simulink model "test"  (R2014a)
settings: Solver=VariableStepAuto  StartTime=0.0  StopTime=10.0  RelTol=1e-3
settings Model: Creator=costa  LastModifiedBy=rcostado
settings DataIOCC: LimitDataPoints=off  SaveFormat=Dataset
settings OptimizationCC: SimCompilerOptimization=off
settings DebuggingCC: MergeDetectMultiDrivingBlocksExec=error  SolverPrmCheckMsg=none  FrameProcessingCompatibilityMsg=error
settings HardwareCC: ProdBitPerPointer=64  ProdLargestAtomicFloat=Float  ProdIntDivRoundTo=Zero  ProdEndianess=LittleEndian  ProdWordSize=64  ProdHWDeviceType=Intel->x86-64 (Windows64)
settings ModelReferenceCC: PropagateSignalLabelsOutOfModel=on
settings RTWCC: RTWCompilerOptimization=off
settings ConfigComp: CovMetricSettings=dw  CovHtmlReporting=on  CovSaveCumulativeToWorkspaceVar=on  CovSaveSingleToWorkspaceVar=on  CovExternalEMLEnable=off

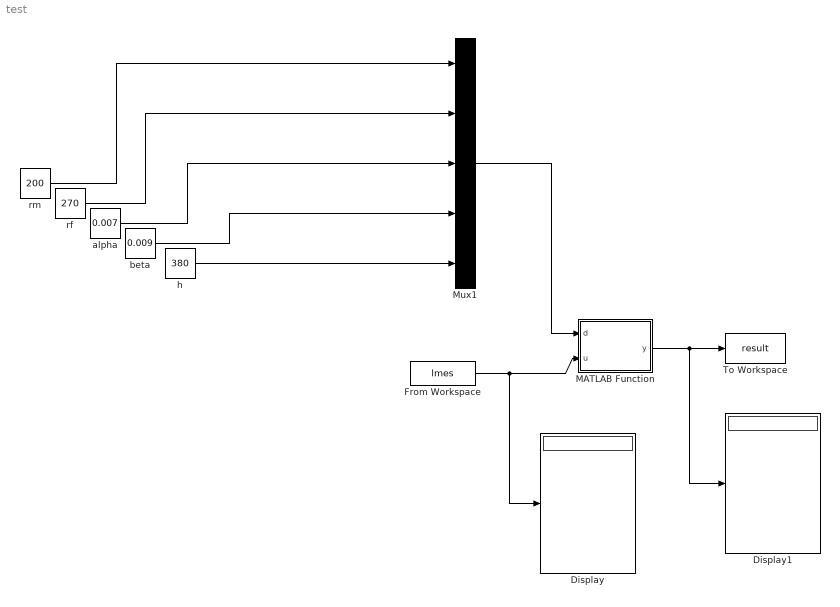
== system test ==
  Display : Display
  Display1 : Display
  From Workspace : FromWorkspace  VariableName=lmes  OutDataTypeStr=double  SampleTime=1
  MATLAB Function : MATLAB Function  TreatAsAtomicUnit=on
  Mux1 : Mux  Inputs=5
  To Workspace : ToWorkspace  VariableName=result  SampleTime=0.01
      settings: Save2DSignal=2-D array (concatenate along first dimension)
  alpha : Constant  Value=0.007
  beta : Constant  Value=0.009
  h : Constant  Value=380
  rf : Constant  Value=270
  rm : Constant  Value=200
  wires:
  From Workspace/1 -> Display/1, MATLAB Function/2(u)
  Mux1/1 -> MATLAB Function/1(d)
  rm/1 -> Mux1/1
  rf/1 -> Mux1/2
  alpha/1 -> Mux1/3
  beta/1 -> Mux1/4
  h/1 -> Mux1/5
  MATLAB Function/1(y) -> Display1/1, To Workspace/1

== matlab function test/MATLAB Function ==
  data: y output; x input; d input; u input
function y = ex1(x,d,u) %#codegen
coder.extrinsic('mysolve');
x0 = x;
y1 = zeros(size(x0));
y1 = mysolve(x0,d,u);
y = y1;

== matlab function test/MATLAB Function ==
  data: y output; d input; u input
function y = ex1(d,u) %#codegen
coder.extrinsic('mysolve');
x0 = [0,0,0,0,0,0];
y1 = zeros(size(x0));
y1 = mysolve(x0,d,u);
y = y1;
